simulink model "HSX_quatro_fin"  (R2023b)
settings: Solver=VariableStepAuto  StartTime=0.0  StopTime=T_end  RelTol=1e-3
values from neighbouring files (symbols this model uses):
  Kaa = 0    [fin.m]
  Kanti = 0.95    [fin.m]
  Ki = K*Rtot    (= 45.48)    [fin.m]
  Kii = 0.001    [fin.m]
  Kp = K*Ltot    (= 10.10125)    [fin.m]
  Kpp = 0.01    [fin.m]
  Lc = 100e-6    (= 0.0001)    [fin.m]
  LHSX = 0.02    [fin.m]
  Limit = 0.999    [fin.m]
  multi_enable = 1    [fin.m]
  n = 4    [fin.m]
  Ra = 0.0096    [fin.m]
  RHSX = 0.09    [fin.m]
  T_hold = 1.5    [fin.m]
  T_trigger = 15    [fin.m]
  Tdead = Ts/100    (= 1e-06)    [fin.m]
  Ts = 1/fs    (= 0.0001)    [fin.m]
  Tsamp = 1/fsamp    (= 2e-05)    [fin.m]
  VDC = 40    [fin.m]
  Vf = 3.1    [fin.m]
libraries: spsCurrentMeasurementLib x10, spsVoltageMeasurementLib x8, spsSeriesRLCBranchLib x8, spsMosfetLib x8, spsTriangleGeneratorLib x4, spsDCVoltageSourceLib x4, spsControlledVoltageSourceLib x2, spsDCMachineLib x2, spsGroundLib x2, spsIdealSwitchLib x2, spsDiodeLib x1, sps_lib x1
settings Model: Creator=baik3-ad  LastModifiedBy=baik3-ad

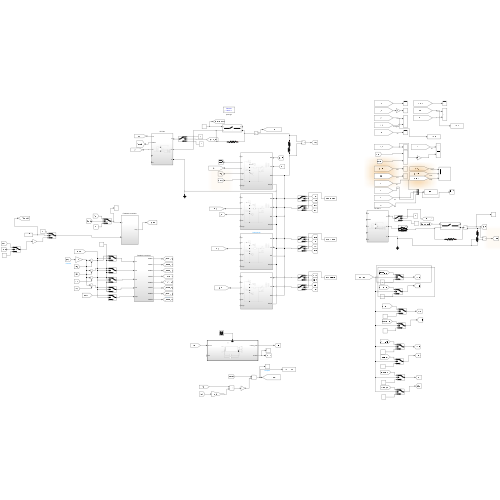
[thumbnail: Simulink's stored preview of the top-level diagram]
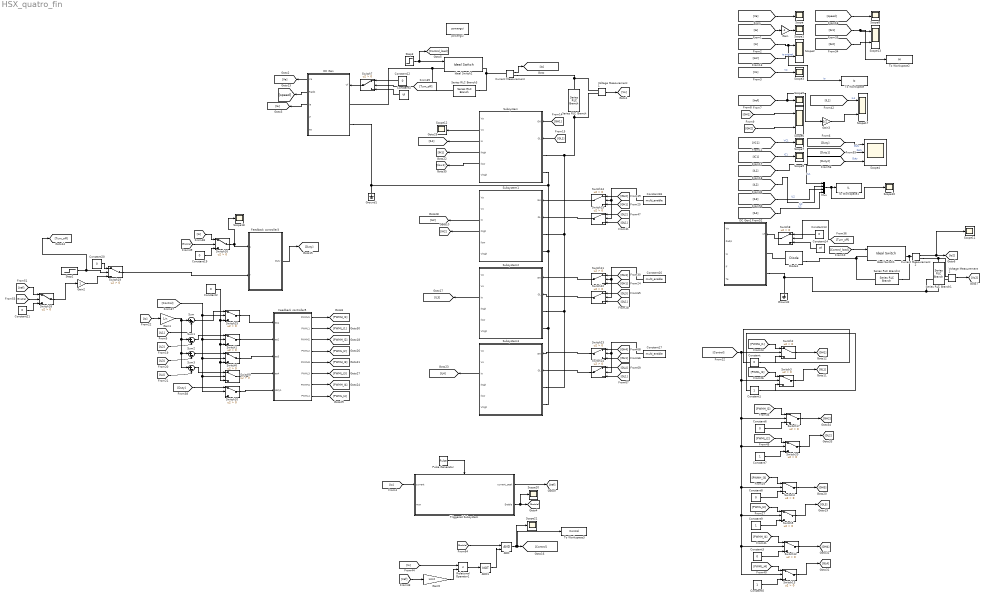
== system HSX_quatro_fin ==
  AND : Logic  IconShape=distinctive  AllPortsSameDT=off  OutDataTypeStr=boolean
  AND1 : Logic  Operator=NOT  IconShape=distinctive  AllPortsSameDT=off  OutDataTypeStr=boolean
  Constant{,2..3,6,8,12..13,19..21} (10 alike) : Constant  Value=0
  Constant{1,5,7,9} (4 alike) : Constant
  Constant14 : Constant  Value=Vf
  Constant16 : Constant  Value=multi_enable
  Constant17 : Constant  Value=multi_enable
  Constant18 : Constant  Value=multi_enable
  Constant4 : Constant  Value=Vf
  Current Measurement : spsCurrentMeasurementLib/Current Measurement  PhasorSimulation=off  OutputType=Complex  PSBequivalent=0
  Current Measurement2 : spsCurrentMeasurementLib/Current Measurement  PhasorSimulation=off  OutputType=Complex  PSBequivalent=0
  DC Gen : Subsystem
  DC Gen1 : Subsystem
  Diode1 : spsDiodeLib/Diode  Ron=0.001  Lon=0  Vf=0.8  IC=0  UseSnubber=0  Rs=500  Cs=250e-9  Measurements=on
  Feedback controller3 : Subsystem
  Feedback controller5 : Subsystem
  Gain : Gain  Gain=-1
  Gain1 : Gain  Gain=1/n
  Gain2 : Gain
  Gain3 : Gain  Gain=1/2
  Gain5 : Gain  Gain=Limit
  Ground1 : spsGroundLib/Ground  LConnTagsString=a
  Ground2 : spsGroundLib/Ground  LConnTagsString=a
  Ideal Switch1 : spsIdealSwitchLib/Ideal Switch  Ron=1e-6  Lon=0  IC=0  Rs=1e8  Cs=0  Measurements=on
  Ideal Switch2 : spsIdealSwitchLib/Ideal Switch  Ron=1e-6  Lon=0  IC=0  Rs=1e8  Cs=0  Measurements=on
  Mux : Mux
  Pulse Generator : DiscretePulseGenerator  PulseType=Time based  Period=Ts  PulseWidth=50
  Relational Operator1 : RelationalOperator  Operator=<  OutDataTypeStr=boolean  RndMeth=Simplest  InputSameDT=off
  Scope{,1,3,5,7..12,18,20..21} (13 alike) : Scope
  Scope{2,6,13,17} (4 alike) : Scope  NumInputPorts=2
  Scope4 : Scope  NumInputPorts=3
  Series RLC Branch : spsSeriesRLCBranchLib/Series RLC Branch  LConnTagsString=__new0  RConnTagsString=__new0  BranchType=RL  Resistance=RHSX*10  Inductance=LHSX*10  SetiL0=off  InitialCurrent=0  Capacitance=1e-6  Setx0=off  InitialVoltage=0  Measurements=None
  Series RLC Branch1 : spsSeriesRLCBranchLib/Series RLC Branch  LConnTagsString=__new0  RConnTagsString=__new0  BranchType=RL  Resistance=RHSX*10  Inductance=LHSX*10  SetiL0=off  InitialCurrent=0  Capacitance=1e-6  Setx0=off  InitialVoltage=0  Measurements=None
  Series RLC Branch3 : spsSeriesRLCBranchLib/Series RLC Branch  LConnTagsString=__new0  RConnTagsString=__new0  BranchType=R  Resistance=1e8  Inductance=0  SetiL0=off  InitialCurrent=0  Capacitance=1e-6  Setx0=off  InitialVoltage=0  Measurements=None
  Series RLC Branch4 : spsSeriesRLCBranchLib/Series RLC Branch  LConnTagsString=__new0  RConnTagsString=__new0  BranchType=R  Resistance=1e8  Inductance=0  SetiL0=off  InitialCurrent=0  Capacitance=1e-6  Setx0=off  InitialVoltage=0  Measurements=None
  Step2 : Step  Time=T_trigger+T_hold  SampleTime=0  VectorParams1D=off  ZeroCross=off
  Step3 : Step  Time=T_trigger  SampleTime=0  VectorParams1D=off  ZeroCross=off
  Subsystem : Subsystem
  Subsystem1 : Subsystem
  Subsystem2 : Subsystem
  Subsystem3 : Subsystem
  Sum{,1..3} (4 alike) : Sum  Inputs=|+-
  Switch{1..20,22..25} (24 alike) : Switch  Criteria=u2 > Threshold  SaturateOnIntegerOverflow=off  InputSameDT=off
  To Workspace : ToWorkspace  VariableName=Io  SaveFormat=Timeseries  SampleTime=-1
  To Workspace1 : ToWorkspace  VariableName=IL  SaveFormat=Timeseries  SampleTime=-1
  To Workspace2 : ToWorkspace  VariableName=IH  SaveFormat=Timeseries  SampleTime=-1
  To Workspace3 : ToWorkspace  VariableName=Control  SaveFormat=Timeseries  SampleTime=-1
  Triggered Subsystem : Subsystem  TreatAsAtomicUnit=on
  Voltage Measurement1 : spsVoltageMeasurementLib/Voltage Measurement  PhasorSimulation=off  OutputType=Complex  PSBequivalent=0
  Voltage Measurement2 : spsVoltageMeasurementLib/Voltage Measurement  PhasorSimulation=off  OutputType=Complex  PSBequivalent=0
  powergui : sps_lib/powergui  Priority=1  SimulationMode=Discrete  SampleTime=Tsamp  frequency=60  Iterations=50  frequencyindice=0  Pbase=100e6  ErrMax=1e-4  UnitsV=kV  UnitsW=MW  buscounter=0  FunctionMessages=off  echomessages=off  EnableUseOfTLC=off  CurrentSourceSwitches=off  DisableSnubberDevices=off  DisableRonSwitches=off  DisableVfSwitches=off  DisplayEquations=off  AutomaticDiscreteSolvers=off  SolverType=Tustin/Backward Euler (TBE)  Interpol=off  ExternalGateDelay=off  methode=off  Ts=100  x0status=blocks  SPID=on  SwTol=0  HookPort=off  NonlinearTolerance=1e-4  nMaxIteration=100  ContinueOnMaxIteration=off  RestoreLinks=warning  ResistiveCurrentMeasurement=off  Frange=[0:2:500]  Ylog=off  Xlog=on  ShowGrid=off  save=off  variable=ZData  structure=0  ZoomFFT=off  StartTime=0.0  cycles=1  DisplayStyle=1  fundamental=60  FreqAxis=off  MaxFrequency=1000  frequencyindicesteady=1  RmsSteady=1  display=off
  wires:
  Step3/1 -> [Control_load], Ideal Switch2/1
  Current Measurement/1 -> [Io]
  Voltage Measurement1/1 -> [Vo]
  [Va] -> Scope/1
  [Io] -> To Workspace/1, Scope2/1  "Io"
  [Vo] -> Scope3/1  "Vo"
  [Ia] -> Gain/1
  Gain/1 -> Scope1/1
  [Iref] -> Gain3/1, Scope5/1
  [VC1] -> Scope7/1  "VC1"
  Switch2/1 -> [GH1]
  Switch3/1 -> [GL1]
  [speed] -> Scope8/1
  [IC1] -> Scope9/1  "IC1"
  [IL1] -> Mux/1  "IL1"
  [PWMH_I1] -> Switch2/1
  Constant/1 -> Switch2/3
  [PWML_I1] -> Switch3/1
  Constant1/1 -> Switch3/3
  Current Measurement2/1 -> Scope11/1, [Io2]
  Voltage Measurement2/1 -> [Vo2]
  [Control_load] -> Ideal Switch1/1
  [Io2] -> Scope2/2  "Io original"
  Switch7/1 -> DC Gen/1(Vf)
  Subsystem/3(Io) -> [IL1]
  Subsystem/2(Vo) -> Scope12/1
  DC Gen/3(Ia) -> [Ia]
  DC Gen/1(Va) -> [Va]
  DC Gen/2(Rad/s) -> [speed]
  Switch4/1 -> [GH3]
  Constant9/1 -> Switch5/3
  [PWML_I3] -> Switch5/1
  [PWMH_I3] -> Switch4/1
  Constant8/1 -> Switch4/3
  Switch5/1 -> [GL3]
  [GH1] -> Subsystem/1(GH)
  [IL2] -> Mux/2  "IL2"
  [IH1] -> To Workspace2/1, Scope13/1
  [IH2] -> Scope13/2
  Subsystem/4(Ihigh) -> [IH1]
  Constant4/1 -> Switch7/3
  [Turn_off] -> Switch7/2
  Constant12/1 -> Switch7/1
  Constant13/1 -> Switch8/1
  Constant14/1 -> Switch8/3
  [Turn_off] -> Switch8/2
  Switch8/1 -> DC Gen1/1(Vf)
  Switch14/1 -> Subsystem1/1(GH)
  Subsystem1/3(Io) -> [IL2]
  Subsystem1/4(Ihigh) -> [IH2]
  Pulse Generator/1 -> Triggered Subsystem/Trigger
  [IL1] -> Scope17/1  "IL1"
  Gain3/1 -> Scope17/2
  [Io] -> Triggered Subsystem/1(current)
  Triggered Subsystem/2(Enable) -> Scope20/1, [Enable]
  Switch15/1 -> Subsystem1/2(GL)
  [GL1] -> Subsystem/2(GL)
  [GH1] -> Scope6/1
  [GH2] -> Scope6/2
  [GH2] -> Switch14/1
  [GL2] -> Switch15/1
  [GH1] -> Switch14/3
  [GL1] -> Switch15/3
  Constant18/1 -> Switch15/2, Switch14/2
  [Enable] -> Switch16/2
  [Io] -> Switch16/1
  Switch16/1 -> Feedback controller3/1(y), Scope18/1
  Constant19/1 -> Switch16/3
  Switch19/1 -> Feedback controller3/2(r)
  Feedback controller3/1(Duty) -> [Duty]
  [Duty] -> Scope4/1  "Duty"
  [Duty1] -> Scope4/2  "Duty"
  [Duty2] -> Scope4/3  "Duty"
  Triggered Subsystem/1(current_peak) -> [Iref]
  [Iref] -> Gain5/1
  [Io] -> Relational Operator1/1
  Gain5/1 -> Relational Operator1/2
  Relational Operator1/1 -> AND1/1
  AND1/1 -> AND/2
  [Enable] -> AND/1
  AND/1 -> Scope21/1, To Workspace3/1, [Control]
  Switch11/1 -> Subsystem2/1(GH)
  Switch22/1 -> Subsystem2/2(GL)
  Constant16/1 -> Switch22/2, Switch11/2
  [GH1] -> Switch11/3
  [GH3] -> Switch11/1
  [GL1] -> Switch22/3
  [GL3] -> Switch22/1
  Switch23/1 -> Subsystem3/1(GH)
  Switch24/1 -> Subsystem3/2(GL)
  [GL1] -> Switch24/3
  [GH1] -> Switch23/3
  Constant17/1 -> Switch24/2, Switch23/2
  [GL4] -> Switch24/1
  [GH4] -> Switch23/1
  Subsystem2/3(Io) -> [IL3]
  Subsystem3/3(Io) -> [IL4]
  [Io] -> Gain1/1
  Gain1/1 -> Sum3/1, Sum2/1, Sum1/1, Sum/1
  [IL1] -> Sum/2
  [IL2] -> Sum1/2
  [IL3] -> Sum2/2
  [IL4] -> Sum3/2
  [Control] -> Switch10/2, Switch9/2, Switch6/2, Switch1/2, Switch25/2
  Sum/1 -> Switch25/1
  Sum1/1 -> Switch1/1
  Sum2/1 -> Switch6/1
  Sum3/1 -> Switch9/1
  Constant2/1 -> Switch9/3, Switch6/3, Switch1/3, Switch25/3
  Switch25/1 -> Feedback controller5/1(eo1)
  Switch1/1 -> Feedback controller5/2(eo2)
  Switch6/1 -> Feedback controller5/3(eo3)
  Switch9/1 -> Feedback controller5/4(eo4)
  [Duty] -> Switch10/1
  Switch10/1 -> Feedback controller5/5(duty1)
  Feedback controller5/1(PWMH1) -> [PWMH_I1]
  Feedback controller5/2(PWML1) -> [PWML_I1]
  Feedback controller5/3(PWMH2) -> [PWMH_I2]
  Feedback controller5/4(PWML2) -> [PWML_I2]
  Feedback controller5/5(PWMH3) -> [PWMH_I3]
  Feedback controller5/6(PWML3) -> [PWML_I3]
  Feedback controller5/7(PWMH4) -> [PWMH_I4]
  Feedback controller5/8(PWML4) -> [PWML_I4]
  Switch12/1 -> [GH4]
  [PWML_I4] -> Switch13/1
  Constant5/1 -> Switch13/3
  Switch13/1 -> [GL4]
  [PWMH_I4] -> Switch12/1
  Constant3/1 -> Switch12/3
  Switch17/1 -> [GH2]
  [PWML_I2] -> Switch20/1
  Constant7/1 -> Switch20/3
  Switch20/1 -> [GL2]
  [PWMH_I2] -> Switch17/1
  [Control] -> Switch17/2, Switch20/2, Switch4/2, Switch5/2, Switch13/2, Switch12/2, Switch3/2, Switch2/2
  Constant6/1 -> Switch17/3
  [IL3] -> Mux/3  "IL2"
  [IL4] -> Mux/4  "IL2"
  Mux/1 -> Scope10/1, To Workspace1/1
  Subsystem/5(Ilow) -> [Ilow1]
  Constant20/1 -> Switch19/1
  Step2/1 -> [Turn_off], Switch19/2
  Gain2/1 -> Switch19/3
  [Iref] -> Switch18/1
  Switch18/1 -> Gain2/1
  [Enable] -> Switch18/2
  Constant21/1 -> Switch18/3
  connections:
  DC Gen/LConn2 -- Subsystem3/LConn2 -- Subsystem2/LConn2 -- Subsystem1/LConn2 -- Subsystem/LConn2 -- Ground1/LConn1
  Current Measurement/RConn1 -- Voltage Measurement1/LConn1 -- Series RLC Branch/LConn1
  Current Measurement/LConn1 -- Ideal Switch2/RConn1 -- Series RLC Branch3/LConn1
  Ideal Switch1/LConn1 -- Diode1/RConn1 -- Series RLC Branch4/RConn1
  Ideal Switch1/RConn1 -- Current Measurement2/LConn1 -- Series RLC Branch4/LConn1
  Series RLC Branch1/LConn1 -- Voltage Measurement2/LConn1 -- Current Measurement2/RConn1
  Diode1/LConn1 -- DC Gen1/LConn1
  DC Gen1/LConn2 -- Series RLC Branch1/RConn1 -- Voltage Measurement2/LConn2 -- Ground2/LConn1
  Ideal Switch2/LConn1 -- DC Gen/LConn1 -- Series RLC Branch3/RConn1
  Voltage Measurement1/LConn2 -- Subsystem3/LConn1 -- Subsystem2/LConn1 -- Subsystem1/LConn1 -- Subsystem/LConn1 -- Series RLC Branch/RConn1

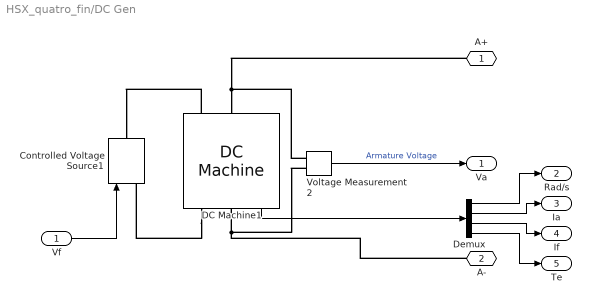
== system HSX_quatro_fin/DC Gen ==
  Vf : Inport
  Controlled Voltage Source1 : spsControlledVoltageSourceLib/Controlled Voltage Source  Initialize=on  Source_Type=DC  Amplitude=0  Phase=0  Frequency=0  Measurements=Voltage
  DC Machine1 : spsDCMachineLib/DC Machine  PresetModel=No  MechanicalLoad=Torque TL  FieldType=Wound  ShowDetailedParameters=on  MeasurementBus=off  RLa="[Ra  0.002]"  RLf=[0.0054 0.0125]  Laf=Laf  MachineConstant=Torque constant (N.m/A)  Ke=1.8  Kt=1.8  J=137  Bm=0  Tf=0  w0=w_initial  Ifinit=0  TsPowergui=0  TsBlock=-1
  Demux : Demux
  Voltage Measurement2 : spsVoltageMeasurementLib/Voltage Measurement  PhasorSimulation=off  OutputType=Complex  PSBequivalent=0
  A+ : PMIOPort  Side=Left
  A- : PMIOPort  Port=2  Side=Left
  Va : Outport
  Rad/s : Outport  Port=2
  Ia : Outport  Port=3
  If : Outport  Port=4
  Te : Outport  Port=5
  wires:
  DC Machine1/1 -> Demux/1
  Vf/1 -> Controlled Voltage Source1/1
  Voltage Measurement2/1 -> Va/1  "Armature Voltage"
  Demux/1 -> Rad/s/1
  Demux/4 -> Te/1
  Demux/3 -> If/1
  Demux/2 -> Ia/1
  connections:
  Voltage Measurement2/LConn1 -- A+/RConn1 -- DC Machine1/LConn1
  A-/RConn1 -- Voltage Measurement2/LConn2 -- DC Machine1/RConn1
  DC Machine1/LConn2 -- Controlled Voltage Source1/RConn1
  DC Machine1/RConn2 -- Controlled Voltage Source1/LConn1

== system HSX_quatro_fin/DC Gen1 ==
  Vf : Inport
  Controlled Voltage Source1 : spsControlledVoltageSourceLib/Controlled Voltage Source  Initialize=on  Source_Type=DC  Amplitude=0  Phase=0  Frequency=0  Measurements=Voltage
  DC Machine1 : spsDCMachineLib/DC Machine  PresetModel=No  MechanicalLoad=Torque TL  FieldType=Wound  ShowDetailedParameters=on  MeasurementBus=off  RLa="[Ra  0.002]"  RLf=[0.0054 0.0125]  Laf=Laf  MachineConstant=Torque constant (N.m/A)  Ke=1.8  Kt=1.8  J=137  Bm=0  Tf=0  w0=w_initial  Ifinit=0  TsPowergui=0  TsBlock=-1
  Demux : Demux
  Voltage Measurement2 : spsVoltageMeasurementLib/Voltage Measurement  PhasorSimulation=off  OutputType=Complex  PSBequivalent=0
  A+ : PMIOPort  Side=Left
  A- : PMIOPort  Port=2  Side=Left
  Va : Outport
  Rad/s : Outport  Port=2
  Ia : Outport  Port=3
  If : Outport  Port=4
  Te : Outport  Port=5
  wires:
  DC Machine1/1 -> Demux/1
  Vf/1 -> Controlled Voltage Source1/1
  Voltage Measurement2/1 -> Va/1  "Armature Voltage"
  Demux/1 -> Rad/s/1
  Demux/4 -> Te/1
  Demux/3 -> If/1
  Demux/2 -> Ia/1
  connections:
  Voltage Measurement2/LConn1 -- A+/RConn1 -- DC Machine1/LConn1
  A-/RConn1 -- Voltage Measurement2/LConn2 -- DC Machine1/RConn1
  DC Machine1/LConn2 -- Controlled Voltage Source1/RConn1
  DC Machine1/RConn2 -- Controlled Voltage Source1/LConn1

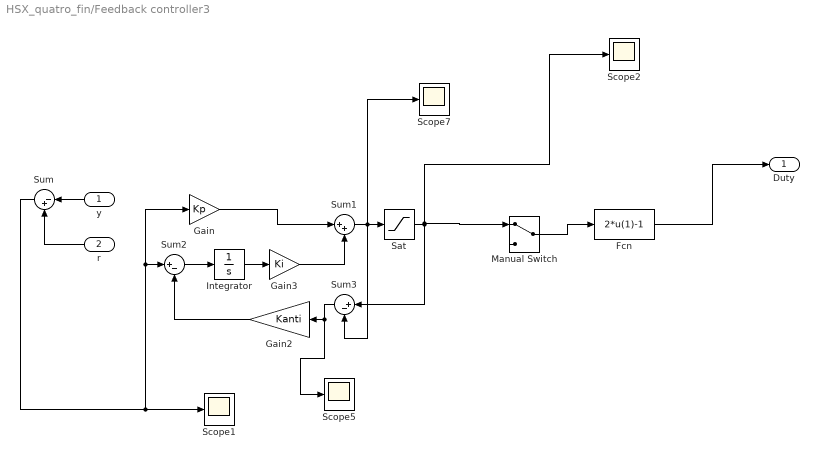
== system HSX_quatro_fin/Feedback controller3 ==
  y : Inport
  r : Inport  Port=2
  Fcn : Fcn  Expr=2*u(1)-1
  Gain : Gain  Gain=Kp
  Gain2 : Gain  Gain=Kanti
  Gain3 : Gain  Gain=Ki
  Integrator : Integrator
  Manual Switch : ManualSwitch
  Sat : Saturate  UpperLimit=1  LowerLimit=0
  Scope{1..2,5,7} (4 alike) : Scope
  Sum : Sum  Inputs=|-+  InputSameDT=on  SaturateOnIntegerOverflow=on  OutDataTypeStr=Inherit: Same as first input
  Sum1 : Sum  Inputs=|++
  Sum2 : Sum  Inputs=|+-
  Sum3 : Sum  Inputs=|+-
  Duty : Outport  VectorParamsAs1DForOutWhenUnconnected=off
  wires:
  Sum/1 -> Scope1/1, Gain/1, Sum2/1
  y/1 -> Sum/1
  r/1 -> Sum/2
  Sat/1 -> Sum3/1, Manual Switch/1, Scope2/1
  Gain/1 -> Sum1/1
  Sum2/1 -> Integrator/1
  Sum3/1 -> Scope5/1, Gain2/1
  Gain2/1 -> Sum2/2
  Integrator/1 -> Gain3/1
  Gain3/1 -> Sum1/2
  Manual Switch/1 -> Fcn/1
  Sum1/1 -> Scope7/1, Sat/1, Sum3/2
  Fcn/1 -> Duty/1

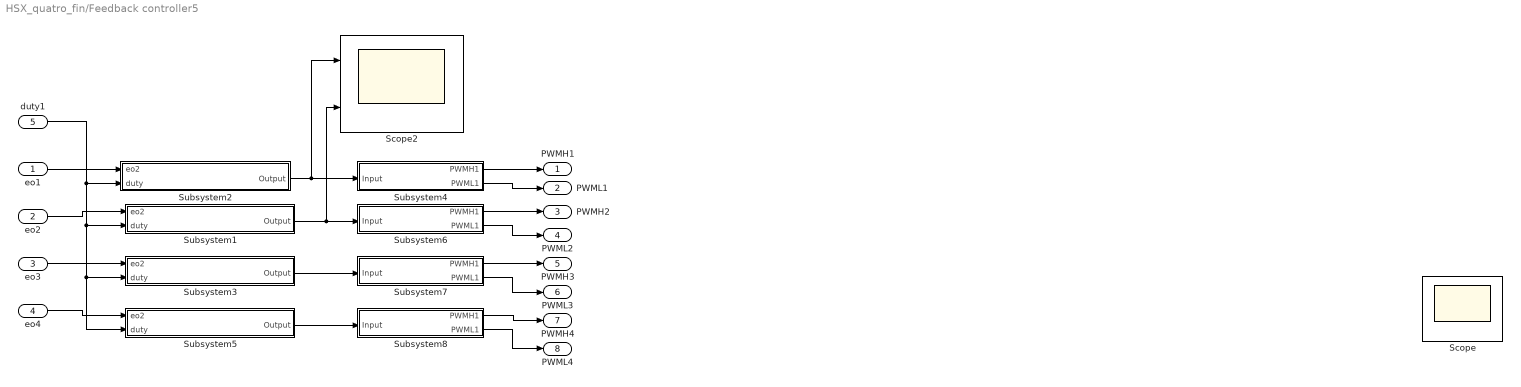
== system HSX_quatro_fin/Feedback controller5 ==
  eo1 : Inport
  eo2 : Inport  Port=2
  eo3 : Inport  Port=3
  eo4 : Inport  Port=4
  duty1 : Inport  Port=5
  Scope : Scope  NumInputPorts=2
  Scope2 : Scope  NumInputPorts=2
  Subsystem1 : Subsystem
  Subsystem2 : Subsystem
  Subsystem3 : Subsystem
  Subsystem4 : Subsystem
  Subsystem5 : Subsystem
  Subsystem6 : Subsystem
  Subsystem7 : Subsystem
  Subsystem8 : Subsystem
  PWMH1 : Outport  VectorParamsAs1DForOutWhenUnconnected=off
  PWML1 : Outport  Port=2  VectorParamsAs1DForOutWhenUnconnected=off
  PWMH2 : Outport  Port=3  VectorParamsAs1DForOutWhenUnconnected=off
  PWML2 : Outport  Port=4  VectorParamsAs1DForOutWhenUnconnected=off
  PWMH3 : Outport  Port=5  VectorParamsAs1DForOutWhenUnconnected=off
  PWML3 : Outport  Port=6  VectorParamsAs1DForOutWhenUnconnected=off
  PWMH4 : Outport  Port=7  VectorParamsAs1DForOutWhenUnconnected=off
  PWML4 : Outport  Port=8  VectorParamsAs1DForOutWhenUnconnected=off
  wires:
  eo1/1 -> Subsystem2/1(eo2)
  eo2/1 -> Subsystem1/1(eo2)
  eo3/1 -> Subsystem3/1(eo2)
  eo4/1 -> Subsystem5/1(eo2)
  duty1/1 -> Subsystem5/2(duty), Subsystem3/2(duty), Subsystem1/2(duty), Subsystem2/2(duty)
  Subsystem2/1(Output) -> Scope2/1, Subsystem4/1(Input)
  Subsystem1/1(Output) -> Scope2/2, Subsystem6/1(Input)
  Subsystem3/1(Output) -> Subsystem7/1(Input)
  Subsystem5/1(Output) -> Subsystem8/1(Input)
  Subsystem4/1(PWMH1) -> PWMH1/1
  Subsystem4/2(PWML1) -> PWML1/1
  Subsystem8/2(PWML1) -> PWML4/1
  Subsystem8/1(PWMH1) -> PWMH4/1
  Subsystem7/2(PWML1) -> PWML3/1
  Subsystem7/1(PWMH1) -> PWMH3/1
  Subsystem6/2(PWML1) -> PWML2/1
  Subsystem6/1(PWMH1) -> PWMH2/1

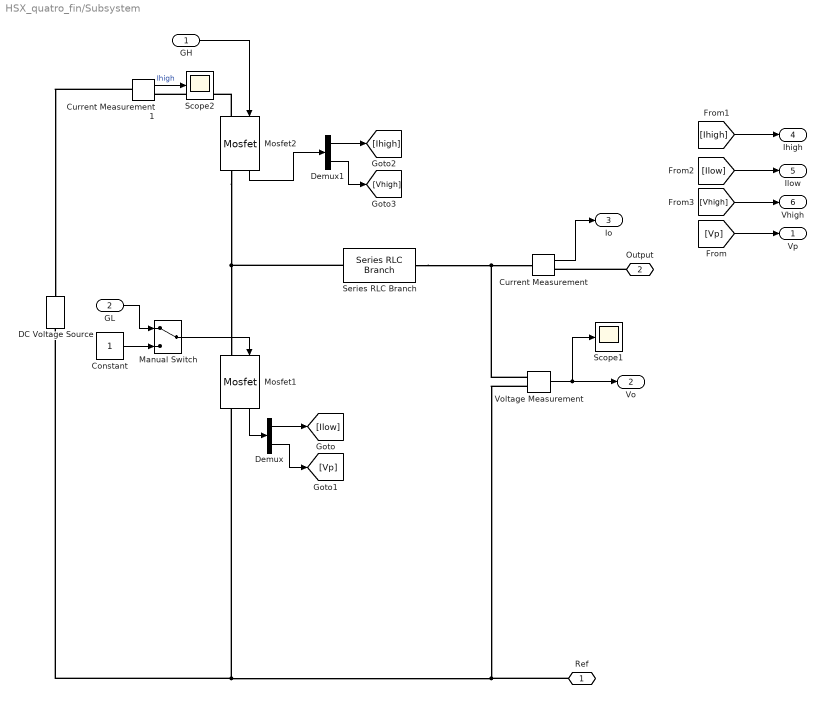
== system HSX_quatro_fin/Subsystem ==
  GH : Inport
  GL : Inport  Port=2
  Constant : Constant
  Current Measurement : spsCurrentMeasurementLib/Current Measurement  PhasorSimulation=off  OutputType=Complex  PSBequivalent=0
  Current Measurement1 : spsCurrentMeasurementLib/Current Measurement  PhasorSimulation=off  OutputType=Complex  PSBequivalent=0
  DC Voltage Source : spsDCVoltageSourceLib/DC Voltage Source  Amplitude=VDC  Measurements=None
  Demux : Demux  Outputs=2
  Demux1 : Demux  Outputs=2
  Manual Switch : ManualSwitch
  Mosfet1 : spsMosfetLib/Mosfet  Ron=0.000001  Lon=0  Rd=0.001  Vfd=0.01  IC=0  Rs=1e5  Cs=inf  Measurements=on
  Mosfet2 : spsMosfetLib/Mosfet  Ron=0.000001  Lon=0  Rd=0.001  Vfd=0.01  IC=0  Rs=1e5  Cs=inf  Measurements=on
  Scope1 : Scope
  Scope2 : Scope
  Series RLC Branch : spsSeriesRLCBranchLib/Series RLC Branch  LConnTagsString=__new0  RConnTagsString=__new0  BranchType=L  Resistance=RHSX*10  Inductance=Lc  SetiL0=off  InitialCurrent=0  Capacitance=1e-6  Setx0=off  InitialVoltage=0  Measurements=None
  Voltage Measurement : spsVoltageMeasurementLib/Voltage Measurement  PhasorSimulation=off  OutputType=Complex  PSBequivalent=0
  Ref : PMIOPort  Side=Left
  Output : PMIOPort  Port=2  Side=Left
  Vp : Outport
  Vo : Outport  Port=2
  Io : Outport  Port=3
  Ihigh : Outport  Port=4
  Ilow : Outport  Port=5
  Vhigh : Outport  Port=6
  wires:
  Voltage Measurement/1 -> Vo/1, Scope1/1
  Manual Switch/1 -> Mosfet1/1
  Current Measurement/1 -> Io/1
  Mosfet1/1 -> Demux/1
  Demux/1 -> [Ilow]
  Demux/2 -> [Vp]
  [Vp] -> Vp/1
  GH/1 -> Mosfet2/1
  Demux1/2 -> [Vhigh]
  Mosfet2/1 -> Demux1/1
  Demux1/1 -> [Ihigh]
  [Ihigh] -> Ihigh/1
  [Ilow] -> Ilow/1
  [Vhigh] -> Vhigh/1
  Current Measurement1/1 -> Scope2/1  "Ihigh"
  Constant/1 -> Manual Switch/2
  GL/1 -> Manual Switch/1
  connections:
  Mosfet2/RConn1 -- Series RLC Branch/LConn1 -- Mosfet1/LConn1
  Voltage Measurement/LConn2 -- DC Voltage Source/LConn1 -- Mosfet1/RConn1 -- Ref/RConn1
  Output/RConn1 -- Current Measurement/RConn1
  Current Measurement1/LConn1 -- DC Voltage Source/RConn1
  Mosfet2/LConn1 -- Current Measurement1/RConn1
  Voltage Measurement/LConn1 -- Current Measurement/LConn1 -- Series RLC Branch/RConn1

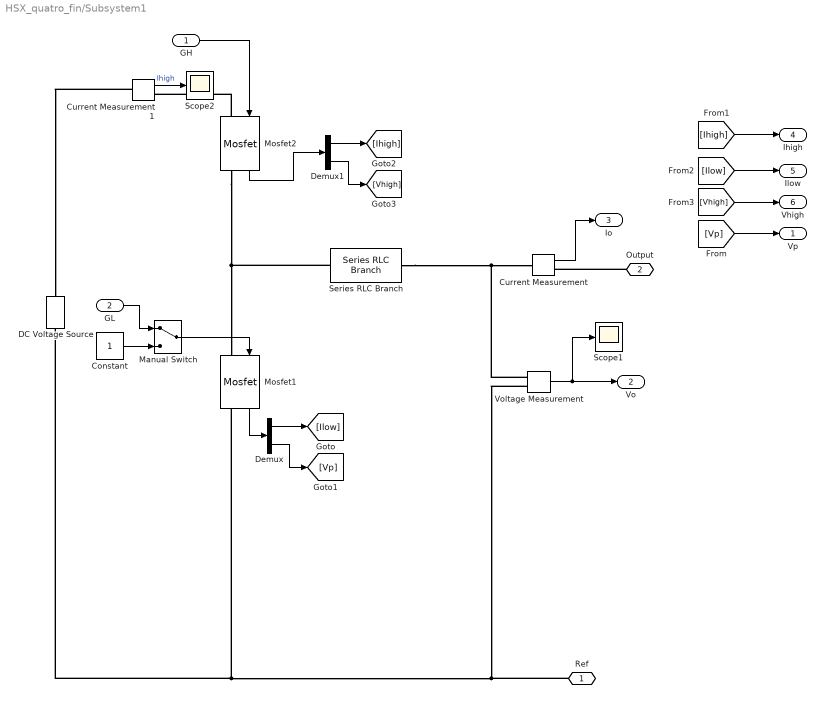
== system HSX_quatro_fin/Subsystem1 ==
  GH : Inport
  GL : Inport  Port=2
  Constant : Constant
  Current Measurement : spsCurrentMeasurementLib/Current Measurement  PhasorSimulation=off  OutputType=Complex  PSBequivalent=0
  Current Measurement1 : spsCurrentMeasurementLib/Current Measurement  PhasorSimulation=off  OutputType=Complex  PSBequivalent=0
  DC Voltage Source : spsDCVoltageSourceLib/DC Voltage Source  Amplitude=VDC  Measurements=None
  Demux : Demux  Outputs=2
  Demux1 : Demux  Outputs=2
  Manual Switch : ManualSwitch
  Mosfet1 : spsMosfetLib/Mosfet  Ron=0.000001  Lon=0  Rd=0.001  Vfd=0.01  IC=0  Rs=1e5  Cs=inf  Measurements=on
  Mosfet2 : spsMosfetLib/Mosfet  Ron=0.000001  Lon=0  Rd=0.001  Vfd=0.01  IC=0  Rs=1e5  Cs=inf  Measurements=on
  Scope1 : Scope
  Scope2 : Scope
  Series RLC Branch : spsSeriesRLCBranchLib/Series RLC Branch  LConnTagsString=__new0  RConnTagsString=__new0  BranchType=L  Resistance=RHSX*10  Inductance=Lc  SetiL0=off  InitialCurrent=0  Capacitance=1e-6  Setx0=off  InitialVoltage=0  Measurements=None
  Voltage Measurement : spsVoltageMeasurementLib/Voltage Measurement  PhasorSimulation=off  OutputType=Complex  PSBequivalent=0
  Ref : PMIOPort  Side=Left
  Output : PMIOPort  Port=2  Side=Left
  Vp : Outport
  Vo : Outport  Port=2
  Io : Outport  Port=3
  Ihigh : Outport  Port=4
  Ilow : Outport  Port=5
  Vhigh : Outport  Port=6
  wires:
  Voltage Measurement/1 -> Vo/1, Scope1/1
  Manual Switch/1 -> Mosfet1/1
  Current Measurement/1 -> Io/1
  Mosfet1/1 -> Demux/1
  Demux/1 -> [Ilow]
  Demux/2 -> [Vp]
  [Vp] -> Vp/1
  GH/1 -> Mosfet2/1
  Demux1/2 -> [Vhigh]
  Mosfet2/1 -> Demux1/1
  Demux1/1 -> [Ihigh]
  [Ihigh] -> Ihigh/1
  [Ilow] -> Ilow/1
  [Vhigh] -> Vhigh/1
  Current Measurement1/1 -> Scope2/1  "Ihigh"
  Constant/1 -> Manual Switch/2
  GL/1 -> Manual Switch/1
  connections:
  Mosfet2/RConn1 -- Series RLC Branch/LConn1 -- Mosfet1/LConn1
  Voltage Measurement/LConn2 -- DC Voltage Source/LConn1 -- Mosfet1/RConn1 -- Ref/RConn1
  Output/RConn1 -- Current Measurement/RConn1
  Current Measurement1/LConn1 -- DC Voltage Source/RConn1
  Mosfet2/LConn1 -- Current Measurement1/RConn1
  Voltage Measurement/LConn1 -- Series RLC Branch/RConn1 -- Current Measurement/LConn1

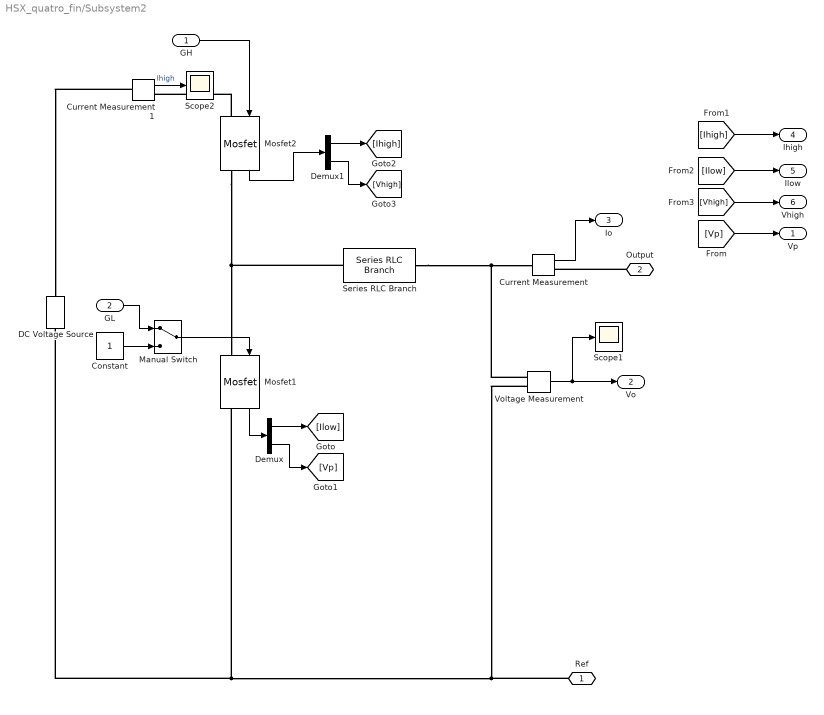
== system HSX_quatro_fin/Subsystem2 ==
  GH : Inport
  GL : Inport  Port=2
  Constant : Constant
  Current Measurement : spsCurrentMeasurementLib/Current Measurement  PhasorSimulation=off  OutputType=Complex  PSBequivalent=0
  Current Measurement1 : spsCurrentMeasurementLib/Current Measurement  PhasorSimulation=off  OutputType=Complex  PSBequivalent=0
  DC Voltage Source : spsDCVoltageSourceLib/DC Voltage Source  Amplitude=VDC  Measurements=None
  Demux : Demux  Outputs=2
  Demux1 : Demux  Outputs=2
  Manual Switch : ManualSwitch
  Mosfet1 : spsMosfetLib/Mosfet  Ron=0.000001  Lon=0  Rd=0.001  Vfd=0.01  IC=0  Rs=1e5  Cs=inf  Measurements=on
  Mosfet2 : spsMosfetLib/Mosfet  Ron=0.000001  Lon=0  Rd=0.001  Vfd=0.01  IC=0  Rs=1e5  Cs=inf  Measurements=on
  Scope1 : Scope
  Scope2 : Scope
  Series RLC Branch : spsSeriesRLCBranchLib/Series RLC Branch  LConnTagsString=__new0  RConnTagsString=__new0  BranchType=L  Resistance=RHSX*10  Inductance=Lc  SetiL0=off  InitialCurrent=0  Capacitance=1e-6  Setx0=off  InitialVoltage=0  Measurements=None
  Voltage Measurement : spsVoltageMeasurementLib/Voltage Measurement  PhasorSimulation=off  OutputType=Complex  PSBequivalent=0
  Ref : PMIOPort  Side=Left
  Output : PMIOPort  Port=2  Side=Left
  Vp : Outport
  Vo : Outport  Port=2
  Io : Outport  Port=3
  Ihigh : Outport  Port=4
  Ilow : Outport  Port=5
  Vhigh : Outport  Port=6
  wires:
  Voltage Measurement/1 -> Vo/1, Scope1/1
  Manual Switch/1 -> Mosfet1/1
  Current Measurement/1 -> Io/1
  Mosfet1/1 -> Demux/1
  Demux/1 -> [Ilow]
  Demux/2 -> [Vp]
  [Vp] -> Vp/1
  GH/1 -> Mosfet2/1
  Demux1/2 -> [Vhigh]
  Mosfet2/1 -> Demux1/1
  Demux1/1 -> [Ihigh]
  [Ihigh] -> Ihigh/1
  [Ilow] -> Ilow/1
  [Vhigh] -> Vhigh/1
  Current Measurement1/1 -> Scope2/1  "Ihigh"
  Constant/1 -> Manual Switch/2
  GL/1 -> Manual Switch/1
  connections:
  Mosfet2/RConn1 -- Series RLC Branch/LConn1 -- Mosfet1/LConn1
  Voltage Measurement/LConn2 -- DC Voltage Source/LConn1 -- Mosfet1/RConn1 -- Ref/RConn1
  Output/RConn1 -- Current Measurement/RConn1
  Current Measurement1/LConn1 -- DC Voltage Source/RConn1
  Mosfet2/LConn1 -- Current Measurement1/RConn1
  Voltage Measurement/LConn1 -- Current Measurement/LConn1 -- Series RLC Branch/RConn1

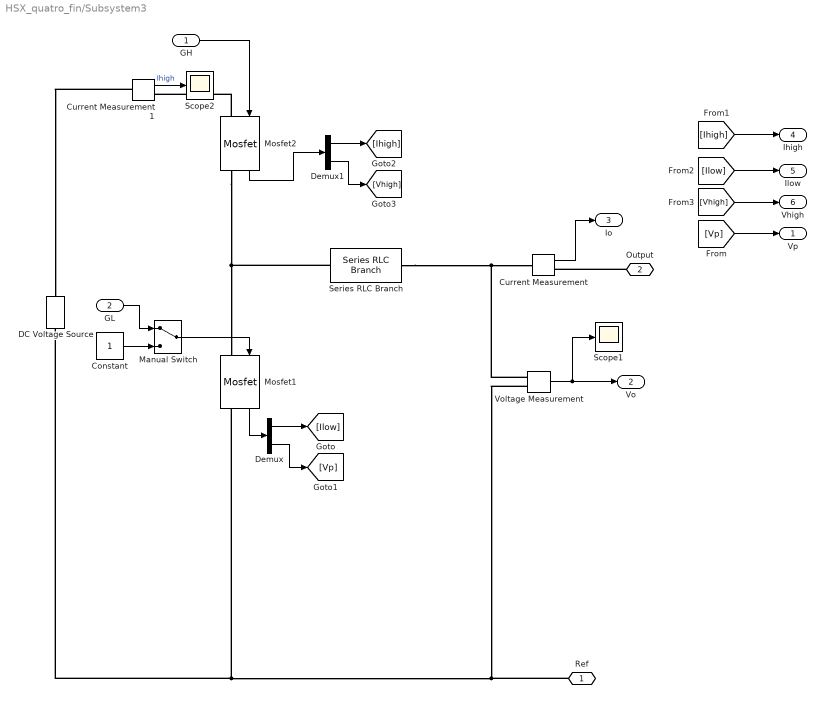
== system HSX_quatro_fin/Subsystem3 ==
  GH : Inport
  GL : Inport  Port=2
  Constant : Constant
  Current Measurement : spsCurrentMeasurementLib/Current Measurement  PhasorSimulation=off  OutputType=Complex  PSBequivalent=0
  Current Measurement1 : spsCurrentMeasurementLib/Current Measurement  PhasorSimulation=off  OutputType=Complex  PSBequivalent=0
  DC Voltage Source : spsDCVoltageSourceLib/DC Voltage Source  Amplitude=VDC  Measurements=None
  Demux : Demux  Outputs=2
  Demux1 : Demux  Outputs=2
  Manual Switch : ManualSwitch
  Mosfet1 : spsMosfetLib/Mosfet  Ron=0.000001  Lon=0  Rd=0.001  Vfd=0.01  IC=0  Rs=1e5  Cs=inf  Measurements=on
  Mosfet2 : spsMosfetLib/Mosfet  Ron=0.000001  Lon=0  Rd=0.001  Vfd=0.01  IC=0  Rs=1e5  Cs=inf  Measurements=on
  Scope1 : Scope
  Scope2 : Scope
  Series RLC Branch : spsSeriesRLCBranchLib/Series RLC Branch  LConnTagsString=__new0  RConnTagsString=__new0  BranchType=L  Resistance=RHSX*10  Inductance=Lc  SetiL0=off  InitialCurrent=0  Capacitance=1e-6  Setx0=off  InitialVoltage=0  Measurements=None
  Voltage Measurement : spsVoltageMeasurementLib/Voltage Measurement  PhasorSimulation=off  OutputType=Complex  PSBequivalent=0
  Ref : PMIOPort  Side=Left
  Output : PMIOPort  Port=2  Side=Left
  Vp : Outport
  Vo : Outport  Port=2
  Io : Outport  Port=3
  Ihigh : Outport  Port=4
  Ilow : Outport  Port=5
  Vhigh : Outport  Port=6
  wires:
  Voltage Measurement/1 -> Vo/1, Scope1/1
  Manual Switch/1 -> Mosfet1/1
  Current Measurement/1 -> Io/1
  Mosfet1/1 -> Demux/1
  Demux/1 -> [Ilow]
  Demux/2 -> [Vp]
  [Vp] -> Vp/1
  GH/1 -> Mosfet2/1
  Demux1/2 -> [Vhigh]
  Mosfet2/1 -> Demux1/1
  Demux1/1 -> [Ihigh]
  [Ihigh] -> Ihigh/1
  [Ilow] -> Ilow/1
  [Vhigh] -> Vhigh/1
  Current Measurement1/1 -> Scope2/1  "Ihigh"
  Constant/1 -> Manual Switch/2
  GL/1 -> Manual Switch/1
  connections:
  Mosfet2/RConn1 -- Series RLC Branch/LConn1 -- Mosfet1/LConn1
  Voltage Measurement/LConn2 -- DC Voltage Source/LConn1 -- Mosfet1/RConn1 -- Ref/RConn1
  Output/RConn1 -- Current Measurement/RConn1
  Current Measurement1/LConn1 -- DC Voltage Source/RConn1
  Mosfet2/LConn1 -- Current Measurement1/RConn1
  Voltage Measurement/LConn1 -- Series RLC Branch/RConn1 -- Current Measurement/LConn1

== system HSX_quatro_fin/Triggered Subsystem ==
  current : Inport
  max : Inport  Port=2
  Trigger : TriggerPort  TriggerType=either  VariantControl=(inherit)
  MATLAB Function : MATLAB Function  TreatAsAtomicUnit=on
  Scope : Scope
  Unit Delay : UnitDelay  SampleTime=-1  HasFrameUpgradeWarning=on
  Unit Delay1 : UnitDelay  SampleTime=-1  HasFrameUpgradeWarning=on
  current_peak : Outport
  Enable : Outport  Port=2
  wires:
  current/1 -> MATLAB Function/1(current)
  Unit Delay/1 -> MATLAB Function/2(peak)
  max/1 -> MATLAB Function/4(max)
  MATLAB Function/1(current_peak) -> current_peak/1, Unit Delay/1
  MATLAB Function/2(enable) -> Enable/1, Unit Delay1/1, Scope/1
  Unit Delay1/1 -> MATLAB Function/3(enable_delay)

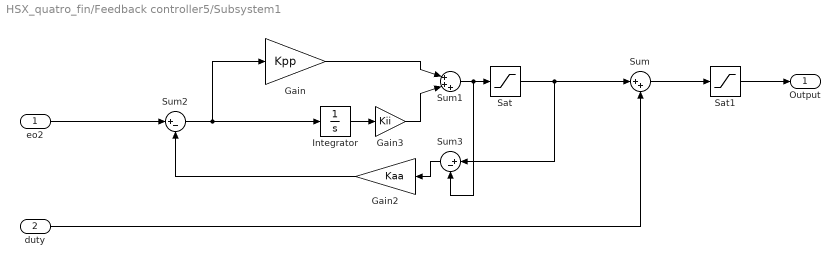
== system HSX_quatro_fin/Feedback controller5/Subsystem1 ==
  eo2 : Inport
  duty : Inport  Port=2
  Gain : Gain  Gain=Kpp
  Gain2 : Gain  Gain=Kaa
  Gain3 : Gain  Gain=Kii
  Integrator : Integrator
  Sat : Saturate  UpperLimit=1  LowerLimit=-1
  Sat1 : Saturate  UpperLimit=1  LowerLimit=0
  Sum : Sum  Inputs=|++
  Sum1 : Sum  Inputs=|+++
  Sum2 : Sum  Inputs=|+-
  Sum3 : Sum  Inputs=|+-
  Output : Outport
  wires:
  Sum1/1 -> Sum3/2, Sat/1
  Gain3/1 -> Sum1/2
  Gain2/1 -> Sum2/2
  Sum2/1 -> Gain/1, Integrator/1
  Sum3/1 -> Gain2/1
  Gain/1 -> Sum1/1
  Integrator/1 -> Gain3/1
  eo2/1 -> Sum2/1
  Sat/1 -> Sum/1, Sum3/1
  duty/1 -> Sum/2
  Sum/1 -> Sat1/1
  Sat1/1 -> Output/1

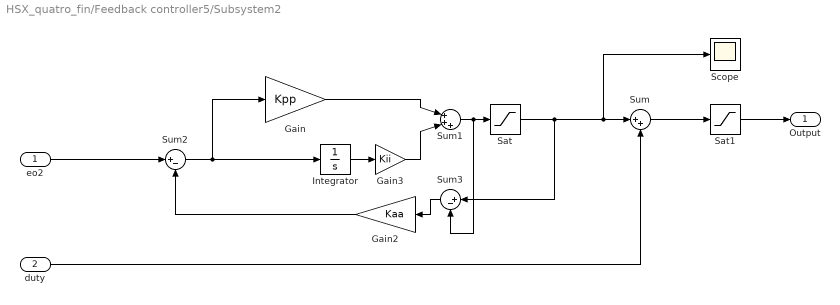
== system HSX_quatro_fin/Feedback controller5/Subsystem2 ==
  eo2 : Inport
  duty : Inport  Port=2
  Gain : Gain  Gain=Kpp
  Gain2 : Gain  Gain=Kaa
  Gain3 : Gain  Gain=Kii
  Integrator : Integrator
  Sat : Saturate  UpperLimit=1  LowerLimit=-1
  Sat1 : Saturate  UpperLimit=1  LowerLimit=0
  Scope : Scope
  Sum : Sum  Inputs=|++
  Sum1 : Sum  Inputs=|+++
  Sum2 : Sum  Inputs=|+-
  Sum3 : Sum  Inputs=|+-
  Output : Outport
  wires:
  Sum1/1 -> Sum3/2, Sat/1
  Gain3/1 -> Sum1/2
  Gain2/1 -> Sum2/2
  Sum2/1 -> Gain/1, Integrator/1
  Sum3/1 -> Gain2/1
  Gain/1 -> Sum1/1
  Integrator/1 -> Gain3/1
  eo2/1 -> Sum2/1
  Sat/1 -> Scope/1, Sum/1, Sum3/1
  duty/1 -> Sum/2
  Sum/1 -> Sat1/1
  Sat1/1 -> Output/1

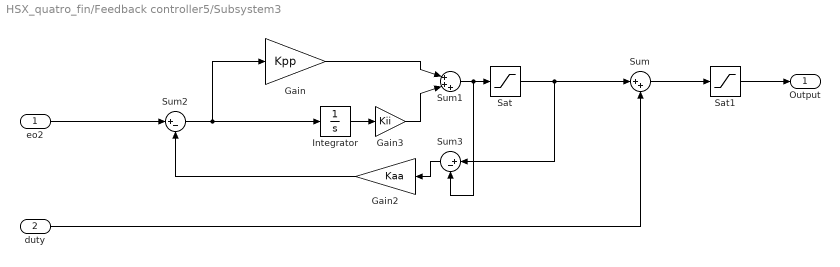
== system HSX_quatro_fin/Feedback controller5/Subsystem3 ==
  eo2 : Inport
  duty : Inport  Port=2
  Gain : Gain  Gain=Kpp
  Gain2 : Gain  Gain=Kaa
  Gain3 : Gain  Gain=Kii
  Integrator : Integrator
  Sat : Saturate  UpperLimit=1  LowerLimit=-1
  Sat1 : Saturate  UpperLimit=1  LowerLimit=0
  Sum : Sum  Inputs=|++
  Sum1 : Sum  Inputs=|+++
  Sum2 : Sum  Inputs=|+-
  Sum3 : Sum  Inputs=|+-
  Output : Outport
  wires:
  Sum1/1 -> Sum3/2, Sat/1
  Gain3/1 -> Sum1/2
  Gain2/1 -> Sum2/2
  Sum2/1 -> Gain/1, Integrator/1
  Sum3/1 -> Gain2/1
  Gain/1 -> Sum1/1
  Integrator/1 -> Gain3/1
  eo2/1 -> Sum2/1
  Sat/1 -> Sum/1, Sum3/1
  duty/1 -> Sum/2
  Sum/1 -> Sat1/1
  Sat1/1 -> Output/1

== system HSX_quatro_fin/Feedback controller5/Subsystem4 ==
  Input : Inport
  AND : Logic  IconShape=distinctive  AllPortsSameDT=off  OutDataTypeStr=boolean
  Delay1 : Delay  DelayLength=1  InitialCondition=0  SampleTime=Tdead
  Fcn : Fcn  Expr=2*u(1)-1
  NOR : Logic  Operator=NOR  IconShape=distinctive  AllPortsSameDT=off
  Relational Operator : RelationalOperator  Operator=>  OutDataTypeStr=boolean  RndMeth=Simplest  InputSameDT=off
  Scope : Scope  NumInputPorts=2
  Scope3 : Scope
  Scope6 : Scope
  Triangle Generator : spsTriangleGeneratorLib/Triangle Generator  Freq=1/Ts  Phase=0  Ts=Tsamp
  PWMH1 : Outport  VectorParamsAs1DForOutWhenUnconnected=off
  PWML1 : Outport  Port=2  VectorParamsAs1DForOutWhenUnconnected=off
  wires:
  AND/1 -> PWMH1/1, Scope/1  "GH"
  Input/1 -> Fcn/1
  Delay1/1 -> NOR/1, AND/2
  Fcn/1 -> Scope3/1, Relational Operator/1
  Triangle Generator/1 -> Scope6/1, Relational Operator/2
  Relational Operator/1 -> Delay1/1, NOR/2, AND/1
  NOR/1 -> PWML1/1, Scope/2  "PWML"

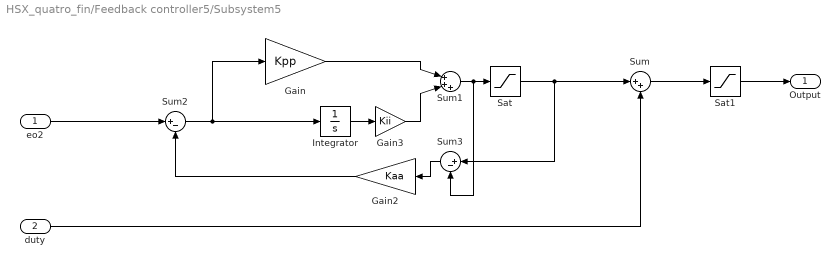
== system HSX_quatro_fin/Feedback controller5/Subsystem5 ==
  eo2 : Inport
  duty : Inport  Port=2
  Gain : Gain  Gain=Kpp
  Gain2 : Gain  Gain=Kaa
  Gain3 : Gain  Gain=Kii
  Integrator : Integrator
  Sat : Saturate  UpperLimit=1  LowerLimit=-1
  Sat1 : Saturate  UpperLimit=1  LowerLimit=0
  Sum : Sum  Inputs=|++
  Sum1 : Sum  Inputs=|+++
  Sum2 : Sum  Inputs=|+-
  Sum3 : Sum  Inputs=|+-
  Output : Outport
  wires:
  Sum1/1 -> Sum3/2, Sat/1
  Gain3/1 -> Sum1/2
  Gain2/1 -> Sum2/2
  Sum2/1 -> Gain/1, Integrator/1
  Sum3/1 -> Gain2/1
  Gain/1 -> Sum1/1
  Integrator/1 -> Gain3/1
  eo2/1 -> Sum2/1
  Sat/1 -> Sum/1, Sum3/1
  duty/1 -> Sum/2
  Sum/1 -> Sat1/1
  Sat1/1 -> Output/1

== system HSX_quatro_fin/Feedback controller5/Subsystem6 ==
  Input : Inport
  AND : Logic  IconShape=distinctive  AllPortsSameDT=off  OutDataTypeStr=boolean
  Delay1 : Delay  DelayLength=1  InitialCondition=0  SampleTime=Tdead
  Fcn : Fcn  Expr=2*u(1)-1
  NOR : Logic  Operator=NOR  IconShape=distinctive  AllPortsSameDT=off
  Relational Operator : RelationalOperator  Operator=>  OutDataTypeStr=boolean  RndMeth=Simplest  InputSameDT=off
  Scope : Scope  NumInputPorts=2
  Scope3 : Scope
  Scope6 : Scope
  Triangle Generator : spsTriangleGeneratorLib/Triangle Generator  Freq=1/Ts  Phase=90  Ts=Tsamp
  PWMH1 : Outport  VectorParamsAs1DForOutWhenUnconnected=off
  PWML1 : Outport  Port=2  VectorParamsAs1DForOutWhenUnconnected=off
  wires:
  AND/1 -> PWMH1/1, Scope/1  "GH"
  Input/1 -> Fcn/1
  Delay1/1 -> NOR/1, AND/2
  Fcn/1 -> Scope3/1, Relational Operator/1
  Triangle Generator/1 -> Scope6/1, Relational Operator/2
  Relational Operator/1 -> Delay1/1, NOR/2, AND/1
  NOR/1 -> PWML1/1, Scope/2  "PWML"

== system HSX_quatro_fin/Feedback controller5/Subsystem7 ==
  Input : Inport
  AND : Logic  IconShape=distinctive  AllPortsSameDT=off  OutDataTypeStr=boolean
  Delay1 : Delay  DelayLength=1  InitialCondition=0  SampleTime=Tdead
  Fcn : Fcn  Expr=2*u(1)-1
  NOR : Logic  Operator=NOR  IconShape=distinctive  AllPortsSameDT=off
  Relational Operator : RelationalOperator  Operator=>  OutDataTypeStr=boolean  RndMeth=Simplest  InputSameDT=off
  Scope : Scope  NumInputPorts=2
  Scope3 : Scope
  Scope6 : Scope
  Triangle Generator : spsTriangleGeneratorLib/Triangle Generator  Freq=1/Ts  Phase=180  Ts=Tsamp
  PWMH1 : Outport  VectorParamsAs1DForOutWhenUnconnected=off
  PWML1 : Outport  Port=2  VectorParamsAs1DForOutWhenUnconnected=off
  wires:
  AND/1 -> PWMH1/1, Scope/1  "GH"
  Input/1 -> Fcn/1
  Delay1/1 -> NOR/1, AND/2
  Fcn/1 -> Scope3/1, Relational Operator/1
  Triangle Generator/1 -> Scope6/1, Relational Operator/2
  Relational Operator/1 -> Delay1/1, NOR/2, AND/1
  NOR/1 -> PWML1/1, Scope/2  "PWML"

== system HSX_quatro_fin/Feedback controller5/Subsystem8 ==
  Input : Inport
  AND : Logic  IconShape=distinctive  AllPortsSameDT=off  OutDataTypeStr=boolean
  Delay1 : Delay  DelayLength=1  InitialCondition=0  SampleTime=Tdead
  Fcn : Fcn  Expr=2*u(1)-1
  NOR : Logic  Operator=NOR  IconShape=distinctive  AllPortsSameDT=off
  Relational Operator : RelationalOperator  Operator=>  OutDataTypeStr=boolean  RndMeth=Simplest  InputSameDT=off
  Scope : Scope  NumInputPorts=2
  Scope3 : Scope
  Scope6 : Scope
  Triangle Generator : spsTriangleGeneratorLib/Triangle Generator  Freq=1/Ts  Phase=270  Ts=Tsamp
  PWMH1 : Outport  VectorParamsAs1DForOutWhenUnconnected=off
  PWML1 : Outport  Port=2  VectorParamsAs1DForOutWhenUnconnected=off
  wires:
  AND/1 -> PWMH1/1, Scope/1  "GH"
  Input/1 -> Fcn/1
  Delay1/1 -> NOR/1, AND/2
  Fcn/1 -> Scope3/1, Relational Operator/1
  Triangle Generator/1 -> Scope6/1, Relational Operator/2
  Relational Operator/1 -> Delay1/1, NOR/2, AND/1
  NOR/1 -> PWML1/1, Scope/2  "PWML"

== matlab function HSX_quatro_fin/Triggered Subsystem/MATLAB Function ==
  data: current input; current_peak output; peak input; enable_delay input; max input; enable output
function [current_peak, enable] = fcn(current,peak,enable_delay, max)
    if current>peak
        current_peak = current;
    else
        current_peak = peak;
    end

    if (max ~= 0)&&(peak>=max)
        current_peak = max;
     
    end
    
    if enable_delay == 1
        enable = 1;
    else

        if current<peak
            enable = 1;
        else
            enable = 0;
        end
    end
